simulink model "EstimateOrientationUsingAHRSandIMU_LSM9DS1"  (R2022a)
settings: Solver=FixedStepAuto  StartTime=0.0  StopTime=inf  RelTol=1e-3
libraries: arduinolib x2, mspfiltlib x1, robotcorelib x1, arduinosensorlib x1
settings Model: ExtModeTrigDuration=2  Creator=The MathWorks, Inc.  LastModifiedBy=cwpan
settings SolverCC: MaxZcPerStep=1
settings OptimizationCC: EnhancedBackFolding=on  PassReuseOutputArgsAs=Individual arguments  ZeroExternalMemoryAtStartup=off  ZeroInternalMemoryAtStartup=off  MaxStackSize=64  OptimizeBlockOrder=speed  DifferentSizesBufferReuse=on  OptimizationCustomize=off  EfficientTunableParamExpr=on
settings DebuggingCC: ParameterPrecisionLossMsg=none  ParameterTunabilityLossMsg=error  UnconnectedInputMsg=warning  UnconnectedOutputMsg=warning  UnconnectedLineMsg=warning
settings HardwareCC: ProdBitPerInt=16  ProdBitPerPointer=16  ProdBitPerSizeT=16  ProdBitPerPtrDiffT=16  ProdLargestAtomicFloat=None  ProdWordSize=8  ProdHWDeviceType=Atmel->AVR  UseEmbeddedCoderFeatures=off  UseSimulinkCoderFeatures=off
settings SFSimCC: MATLABDynamicMemAlloc=off
settings RTWCC: SystemTargetFile=ert.tlc  HardwareBoard=Arduino Uno  TemplateMakefile=ert_default_tmf  Toolchain=Arduino AVR  BuildConfiguration=Faster Runs  DLArmComputeVersion=19.05
settings CodeAppCC: ForceParamTrailComments=on  IgnoreCustomStorageClasses=off  OperatorAnnotations=on  SimulinkDataObjDesc=on  SFDataObjDesc=on  InsertBlockDesc=on
settings ERTTargetCC: SupportContinuousTime=on  SupportNonInlinedSFcns=on  SupportVariableSizeSignals=on  ExtModeStaticAllocSize=250

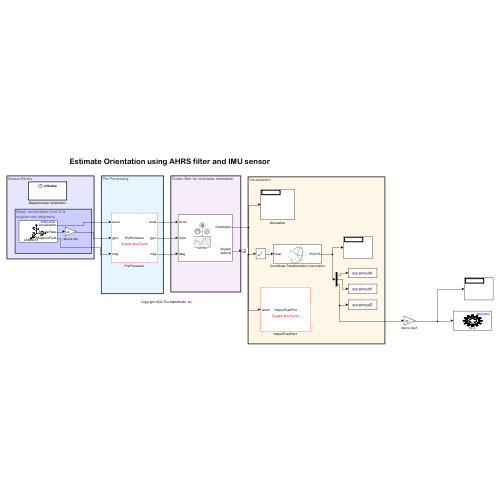
[thumbnail: Simulink's stored preview of the top-level diagram]
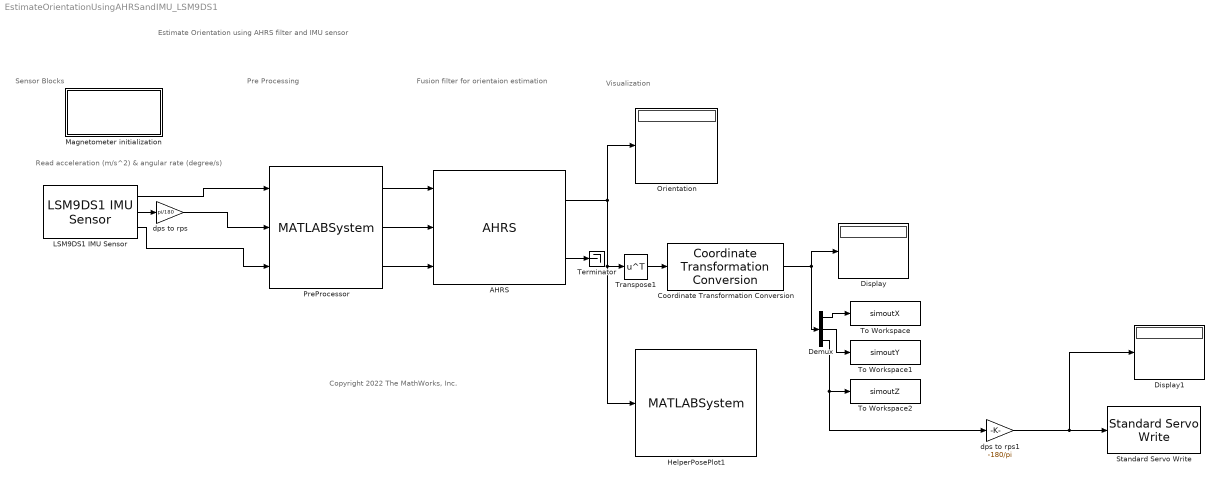
== system EstimateOrientationUsingAHRSandIMU_LSM9DS1 ==
  note: Visualization
  note: Fusion filter for orientaion estimation
  note: Pre Processing
  note: Read  acceleration (m/s^2) &
      | angular rate (degree/s)
  note: Sensor Blocks
  note: Copyright 2022 The MathWorks, Inc.
  note: Estimate Orientation using AHRS filter and IMU sensor
  AHRS : mspfiltlib/AHRS  DispRefFrame=NED  DecimationFactor=1  InitialProcessNoise=ahrsfilter.defaultProcessNoise  OrientationFormat=quaternion  SimulateUsing=Interpreted execution  AccelerometerNoise=0.0001924722  GyroscopeNoise=9.1385e-5  MagnetometerNoise=0.1  GyroscopeDriftNoise=12.0462e-13  LinearAccelerationNoise=0.0096236100000000012  MagneticDisturbanceNoise=0.5  LinearAccelerationDecayFactor=0.5  MagneticDisturbanceDecayFactor=0.5  ExpectedMagneticFieldStrength=50
      settings: SourceProductBaseCode=NV,TF,NV
  Coordinate Transformation Conversion : robotcorelib/Coordinate Transformation Conversion  InputRepresentation=Quaternion  InputEulerSequence=ZYX  ShowTrVecInputPort=on  OutputRepresentation=Euler Angles  OutputEulerSequence=XYZ  ShowTrVecOutputPort=on  SimulateUsing=Interpreted execution
      settings: SourceProductBaseCode=RO,NV,RR,UV
  Demux : Demux  Outputs=3
  Display : Display
  Display1 : Display
  HelperPosePlot1 : MATLABSystem  System=HelperPosePlot  OrientationFormat=Quaternion
      mask Type: HelperPosePlot
      mask Display:
      | disp('HelperPosePlot');
      | port_label('input',1,'orient');
  LSM9DS1 IMU Sensor : arduinosensorlib/LSM9DS1 IMU Sensor  AccelandGyroAddress=0x6B  MagnetometerAddress=0x1E  EnableAccel=on  EnableGyro=on  EnableMag=on  AccelerometerOutputDataRate=119 Hz  AccelerometerFullScaleRange=+/- 2g  AccelerometerBandwidth=50 Hz  GyroscopeOutputDataRate=119 Hz  GyroscopeFullScaleRange=245 dps  GyroscopeBandwidthMode=0  GyroscopeHighPassFilterEnabled=on  GyroscopeHighPassFilterMode=0  MagnetometerOutputDataRate=40 Hz  MagnetometerFullScaleRange=+/- 4 gauss  SampleTime=0.1
      settings: SourceProductBaseCode=ARDUINO
  Magnetometer initialization : Subsystem  TreatAsAtomicUnit=on
  Orientation : Display
  PreProcessor : MATLABSystem  System=PreProcessor  MagOffsets=[-0.184295510626469,0.103537860374665,-0.078136598893169]  AccelXAxisIndex=1  AccelXAxisSign=+  AccelYAxisIndex=2  AccelYAxisSign=+  AccelZAxisIndex=3  AccelZAxisSign=+  GyroXAxisIndex=1  GyroXAxisSign=+  GyroYAxisIndex=2  GyroYAxisSign=+  GyroZAxisIndex=3  GyroZAxisSign=+  MagXAxisIndex=1  MagXAxisSign=+  MagYAxisIndex=2  MagYAxisSign=-  MagZAxisIndex=3  MagZAxisSign=+
      mask Type: PreProcessor
      mask Display:
      | disp('PreProcessor');
      | port_label('input',1,'accel');
      | port_label('input',2,'gyro');
      | port_label('input',3,'mag');
      | port_label('output',1,'accel');
      | port_label('output',2,'gyro');
      | port_label('output',3,'mag');
  Standard Servo Write : arduinolib/Standard Servo Write  pinNumber=4  ServoIndex=0  blockPlatform=arduino
  Terminator : Terminator
  To Workspace : ToWorkspace  VariableName=simoutX  SampleTime=-1
  To Workspace1 : ToWorkspace  VariableName=simoutY  SampleTime=-1
  To Workspace2 : ToWorkspace  VariableName=simoutZ  SaveFormat=Structure  SampleTime=-1
      settings: Save2DSignal=2-D array (concatenate along first dimension)
  Transpose1 : Math  Operator=transpose
  dps to rps : Gain  Gain=pi/180  OutDataTypeStr=double  LockScale=on
  dps to rps1 : Gain  Gain=-180/pi  OutDataTypeStr=double  LockScale=on
  wires:
  PreProcessor/2 -> AHRS/2
  AHRS/2 -> Terminator/1
  PreProcessor/1 -> AHRS/1
  PreProcessor/3 -> AHRS/3
  AHRS/1 -> Transpose1/1, HelperPosePlot1/1, Orientation/1
  LSM9DS1 IMU Sensor/2 -> dps to rps/1
  dps to rps/1 -> PreProcessor/2
  LSM9DS1 IMU Sensor/1 -> PreProcessor/1
  LSM9DS1 IMU Sensor/3 -> PreProcessor/3
  Coordinate Transformation Conversion/1 -> Demux/1, Display/1
  Transpose1/1 -> Coordinate Transformation Conversion/1
  Demux/1 -> To Workspace/1
  Demux/2 -> To Workspace1/1
  Demux/3 -> dps to rps1/1, To Workspace2/1
  dps to rps1/1 -> Display1/1, Standard Servo Write/1

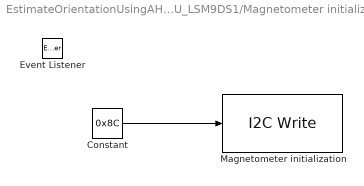
== system EstimateOrientationUsingAHRSandIMU_LSM9DS1/Magnetometer initialization ==
  Constant : Constant  Value=0x8C  OutDataTypeStr=uint8
  Event Listener : EventListener  DisableCoverage=on  EventName=reset
  Magnetometer initialization : arduinolib/I2C Write  Priority=1  I2CModule=0  Mode=Master  SlaveAddress=0x1E  SlaveByteOrder=BigEndian  Direction=Transmitter  RegisterAddressMode=on  RegisterAddress=0x60  SlaveDataType=uint8  DataLength=1  NoAck=off  RepeatedStart=off  OutputStatus=off  blockPlatform=ARDUINO
      settings: SourceProductBaseCode=ARDUINO
  wires:
  Constant/1 -> Magnetometer initialization/1
